simulink model "exampl_Storage_strat_enhanced_R2019a"  (R2019a)
settings: Solver=ode45  StartTime=0.0  StopTime=3*3600-2  RelTol=1e-3  EnableMultiTasking=on
undefined symbols (not defined in the file): path_carnot
libraries: carnot x59, simulink x10
(part 1 of 2)
settings Model: Creator=drhf  LastModifiedBy=P41573
settings DataIOCC: LimitDataPoints=on  SaveFormat=Array  ReturnWorkspaceOutputs=off
settings OptimizationCC: ExpressionDepthLimit=2147483647  LifeSpan=inf
settings DebuggingCC: UnderspecifiedInitializationDetection=Classic  MergeDetectMultiDrivingBlocksExec=none  SolverPrmCheckMsg=warning  StateNameClashWarn=warning  SFUnexpectedBacktrackingDiag=warning  SFNoUnconditionalDefaultTransitionDiag=warning  SFExecutionAtInitializationDiag=none  ArithmeticOperatorsInVariantConditions=warning
settings HardwareCC: ProdBitPerPointer=32  ProdBitPerSizeT=32  ProdBitPerPtrDiffT=32  ProdLargestAtomicFloat=None  ProdIntDivRoundTo=Undefined  ProdEndianess=Unspecified  ProdWordSize=32  ProdHWDeviceType=32-bit Generic
settings ModelReferenceCC: PropagateSignalLabelsOutOfModel=off
settings SFSimCC: SimUseLocalCustomCode=off
settings RTWCC: RTWUseLocalCustomCode=off
settings CodeAppCC: StateflowObjectComments=on
settings GRTTargetCC: TargetLangStandard=C89/C90 (ANSI)  GeneratePreprocessorConditionals=Disable all  CombineOutputUpdateFcns=off  GRTInterface=on
settings ConfigComp: CovMetricSettings=dw  CovHtmlReporting=on  CovSaveCumulativeToWorkspaceVar=on  CovSaveSingleToWorkspaceVar=on  CovExternalEMLEnable=off

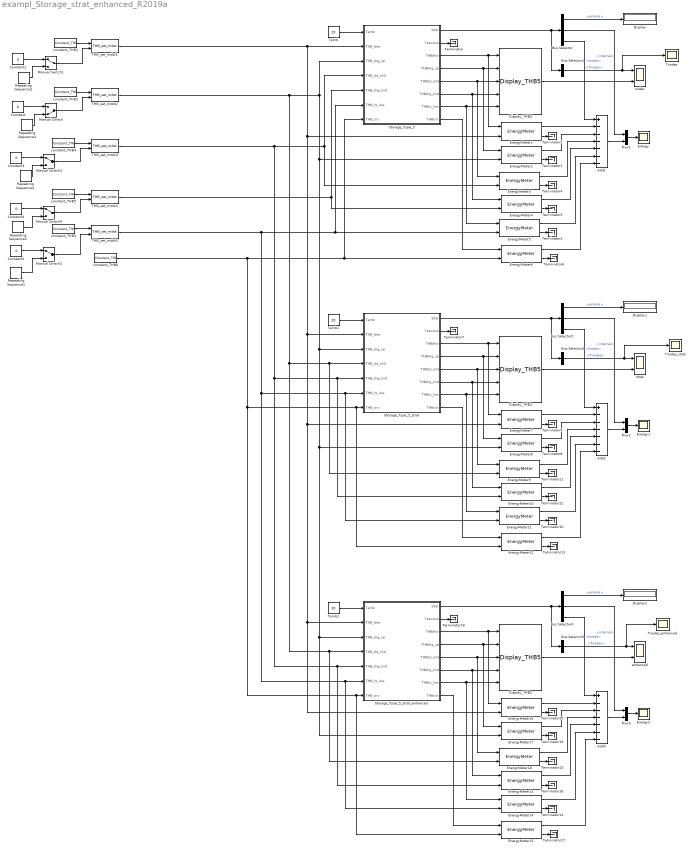
== system exampl_Storage_strat_enhanced_R2019a ==
  Add1 : Sum  Inputs=+------
  Add2 : Sum  Inputs=+------
  Add3 : Sum  Inputs=+------
  Bus Selector : BusSelector  OutputSignals=volume,energy.internal,energy.losses
  Bus Selector1 : BusSelector  OutputSignals=Tnodes
  Bus Selector2 : BusSelector  OutputSignals=volume,energy.internal,energy.losses
  Bus Selector3 : BusSelector  OutputSignals=Tnodes
  Bus Selector4 : BusSelector  OutputSignals=volume,energy.internal,energy.losses
  Bus Selector5 : BusSelector  OutputSignals=Tnodes
  Constant{,1..4} (5 alike) : Constant  Value=0
  Display : Display
  Display1 : Display
  Display2 : Display
  Display_THB1 : carnot/Outputs/Display_THB5  t=off  m=on  p=off  id=off  mix=off  d=off
      settings: SourceProductName=Carnot
  Display_THB2 : carnot/Outputs/Display_THB5  t=off  m=on  p=off  id=off  mix=off  d=off
      settings: SourceProductName=Carnot
  Display_THB5 : carnot/Outputs/Display_THB5  t=off  m=on  p=off  id=off  mix=off  d=off
      settings: SourceProductName=Carnot
  Energy : Scope
  Energy1 : Scope
  Energy2 : Scope
  EnergyMeter{1..18} (18 alike) : carnot/Control/EnergyMeter
      settings: SourceProductName=Carnot
  Manual Switch : ManualSwitch  CurrentSetting=0
  Manual Switch{1..4} (4 alike) : ManualSwitch
  Mux1 : Mux  Inputs=2
  Mux2 : Mux  Inputs=2
  Mux3 : Mux  Inputs=2
  Repeating Sequence1 : simulink/Sources/Repeating Sequence  rep_seq_t=[ 0 3600 3600+eps(3600) 7200 7200+eps(7200) 10800]  rep_seq_y=[ 0.12 0.12 0.11+0*eps(3600) 0.11 0.05+0*eps(7200) 0.05]
  Repeating Sequence2 : simulink/Sources/Repeating Sequence  rep_seq_t=[ 0 3600 3600+eps(3600) 7200 7200+eps(7200) 10440 10440+eps(10440) 11160]  rep_seq_y=[ 0 0 0.05+0*eps(3600) 0.05 0.2+0*eps(7200) 0.2 0+0*eps(10440) 0]
  Repeating Sequence3 : simulink/Sources/Repeating Sequence  rep_seq_t=[ 0 3600 3600+eps(3600) 7200 7200+eps(7200) 10800]  rep_seq_y=[ 0 0 0.1+0*eps(3600) 0.1 0.15+0*eps(7200) 0.15]
  Repeating Sequence4 : simulink/Sources/Repeating Sequence  rep_seq_t=[ 0 3600 3600+eps(3600) 7200 7200+eps(7200) 10800]  rep_seq_y=[ 0.11 0.11 0.1+0*eps(3600) 0.1 0.11+0*eps(7200) 0.11]
  Repeating Sequence5 : simulink/Sources/Repeating Sequence  rep_seq_t=[ 0 3600 3600+eps(3600) 7200 7200+eps(7200) 10800]  rep_seq_y=[ 0.12 0.12 0+0*eps(3600) 0 0.05+0*eps(7200) 0.05]
  Storage_Type_5 : Subsystem  AncestorBlock=carnot/Storage/Thermal/Storage_Type_5  mask(Combi-storage for hot water production and heating){t0=[10:5:55], hgt=1.8108, stgtype=5, tini=[10 15 20 25 30 35 40 45 50 55], mpts=[1 2 3 4 5 6 7 8 9 10], PathName=fullfile(path_carnot('libsl'),'Storage','Thermal','Storage_Type_5','parameter_set'), FileName='<user defined>', userPath=off, userParam=on, uwall=1, ubot=1, utop=1, axcond=1, volume=0.8, dia=0.75, standing=standing cylinder, nodes=10, mpoints=10, Tsensor=[0.2 0.5 0.7], pipe3inlet=1, pipe3outlet=0.6, pipe3dia=0.05, pipe1inlet=0.55, pipe1outlet=0.45, pipe1dia=0.05, hx1inlet=0.4, hx1outlet=0, hx1dia=0.03, hx1uac=200, hx1uam=0.15, hx1uat=0.6, hx1dplin=20, hx1dpqua=20, pipe2inlet=0.45, pipe2outlet=0.55, pipe2dia=0.05, hx2inlet=0, hx2outlet=1, hx2dia=0.025, hx2uac=450, hx2uam=0.4, hx2uat=0.8, hx2dplin=200, hx2dpqua=200, hx3inlet=0.9, hx3outlet=1, hx3dia=0.01, hx3uac=100, hx3uam=0, hx3uat=0, hx3dplin=10, hx3dpqua=10}
      mask prompts: t0 "Initial temperature (vector or scalar) in °C"; hgt "Height of storage in m"; stgtype "Storage Type (0..5)"; tini "Start temperatures of nodes in °C"; mpts "Index to measured nodes"; PathName "Path"; FileName "Parameter set"; userPath "Edit path and name of parameter set"; userParam "User defined parameters"; uwall "Heat transfer coefficient to ambient [W/m²K]"; ubot "Heat transfer coefficient to ambient bottom [W/m²K]"; utop "Heat transfer coefficient to ambient top [W/m²K]"; axcond "Effective thermal conductivity [W/m/K]"; volume "Volume [m³]"; dia "Diameter [m]"; standing "Position"; nodes "Number of nodes"; mpoints "Number of node temperatures (for display)"; Tsensor "Temperature sensor position (0..1, 0 = bottom, 1 = top)"; pipe3inlet "relative height of inlet, range from 0 (= bottom) to 1 (= top)"; pipe3outlet "relative height of outlet, range from 0 (= bottom) to 1 (= top)"; pipe3dia "Diameter of pipe in m"; pipe1inlet "relative height of inlet, range from 0 (= bottom) to 1 (= top)"; pipe1outlet "relative height of outlet, range from 0 (= bottom) to 1 (= top)"; pipe1dia "Diameter of pipe in m"; hx1inlet "relative height of inlet"; hx1outlet "relative height of outlet"; hx1dia "Diameter of HX pipe [m]"; hx1uac "uac: heat transfer coefficient [W/K /(kg/s) /(°C)]"; hx1uam "uam: massflow dependent heat transfer [-]"; hx1uat "uat: temperature difference dependent heat transfer [-]"; hx1dplin "pressure drop linear in mdot [Pa*s/kg]"; hx1dpqua "pressure drop quadratic in mdot [Pa*s²/kg²]"; pipe2inlet "relative height of inlet, range from 0 (= bottom) to 1 (= top)"; pipe2outlet "relative height of outlet, range from 0 (= bottom) to 1 (= top)"; pipe2dia "Diameter of pipe in m"; hx2inlet "relative height of inlet"; hx2outlet "relative height of outlet"; hx2dia "Diameter of HX pipe [m]"; hx2uac "uac: heat transfer coefficient [W/K /(kg/s) /(°C)]"; hx2uam "uam: massflow dependent heat transfer [-]"; hx2uat "uat: temperature difference dependent heat transfer [-]"; hx2dplin "pressure drop linear in mdot [Pa*s/kg]"; hx2dpqua "pressure drop quadratic in mdot [Pa*s²/kg²]"; hx3inlet "relative height of inlet"; hx3outlet "relative height of outlet"; hx3dia "Diameter of HX pipe [m]"; hx3uac "uac: constant heat transfer coefficient [W/K]"; hx3uam "uam: massflow dependent heat transfer [W*s/(K*kg)]"; hx3uat "uat: temperature difference dependent heat transfer [W/K²]"; hx3dplin "Pressure drop coefficient dplin [Pa/(kg/s)]"; hx3dpqua "Pressure drop coefficient dpqua [Pa/(kg/s)²]"
      mask help:
      | Combi-storage for hot water production and heating.  The backup heater for the heating circuit is working on the storage.
      | The storage model has the following components (with their typical position):
      | - one solar heat exchanger (lower part)
      | - one hot water heat exchanger (total height)
      | - one hot water circulation heat exchanger (top part)
      | - one pipe connection for the heating circuit (middle part)
      | - one pipe connection for the backup heater (middle part)
      | - one pipe connection to heat the storage for hot water production (upper part )
      mask init:
      | [ok, param] = CarnotCallbacks_StorageConf('SetParam',stgtype,gcbh,PathName,FileName);
      mask Help: web(fullfile(path_carnot('help'),'Storage_Type_N.html'),'-helpbrowser')
      mask TypeOptions hgt: HX_EN12977_1/hgt | HX_EN12977_2/hgt | HX_EN12977_3/hgt | Pipe_Connection_1/hgt | Pipe_Connection_2_old/hgt | Pipe_Connection_3/hgt | Pipe_Connection_3_enhanced/hgt | Pipe_Connection_3_strat/hgt
      mask TypeOptions stgtype: CreateSdat/stgtype
      mask TypeOptions tini: sfun_storageTnodes/tini
      mask TypeOptions mpts: select_T/Indices
      mask Callback userPath: [ok, param] = CarnotCallbacks_StorageConf('UserEdit',5,gcbh);
      mask Callback userParam: [ok, param] = CarnotCallbacks_StorageConf('UserEdit',5,gcbh);
      mask TypeOptions uwall: sfun_storageTnodes/uloss
      mask TypeOptions ubot: sfun_storageTnodes/ubot
      mask TypeOptions utop: sfun_storageTnodes/utop
      mask TypeOptions axcond: sfun_storageTnodes/cond
      mask TypeOptions volume: sfun_storageTnodes/volume | CreateSdat/volume
      mask TypeOptions dia: sfun_storageTnodes/dia | Pipe_Connection_1/dstg | Pipe_Connection_2_old/dstg | Pipe_Connection_3/dstg | Pipe_Connection_3_strat/dstg
      mask TypeOptions standing: sfun_storageTnodes/standing
      mask TypeOptions nodes: sfun_storageTnodes/nodes | select_T/InputPortWidth | HX_EN12977_1/nodes | HX_EN12977_2/nodes | HX_EN12977_3/nodes | Pipe_Connection_1/nodes | Pipe_Connection_2_old/nodes | Pipe_Connection_3/nodes | Pipe_Connection_3_enhanced/nodes | Pipe_Connection_3_strat/nodes
      mask TypeOptions Tsensor: T_Sensor_Surface/pos
      mask TypeOptions pipe3inlet: Pipe_Connection_3/h_in | Pipe_Connection_3_strat/h_in | Pipe_Connection_3_enhanced/h_in
      mask TypeOptions pipe3outlet: Pipe_Connection_3/h_out | Pipe_Connection_3_enhanced/h_out | Pipe_Connection_3_strat/h_out
      mask TypeOptions pipe3dia: Pipe_Connection_3/dpipe | Pipe_Connection_3_enhanced/dia | Pipe_Connection_3_strat/dpipe
      mask TypeOptions pipe1inlet: Pipe_Connection_1/h_in
      mask TypeOptions pipe1outlet: Pipe_Connection_1/h_out
      mask TypeOptions pipe1dia: Pipe_Connection_1/dpipe
      mask TypeOptions hx1inlet: HX_EN12977_1/h_in
      mask TypeOptions hx1outlet: HX_EN12977_1/h_out
      mask TypeOptions hx1dia: HX_EN12977_1/dia
      mask TypeOptions hx1uac: HX_EN12977_1/ua0
      mask TypeOptions hx1uam: HX_EN12977_1/uam
      mask TypeOptions hx1uat: HX_EN12977_1/uat
      mask TypeOptions hx1dplin: HX_EN12977_1/dplin
      mask TypeOptions hx1dpqua: HX_EN12977_1/dpqua
      mask TypeOptions pipe2inlet: Pipe_Connection_2_old/h_in
      mask TypeOptions pipe2outlet: Pipe_Connection_2_old/h_out
      mask TypeOptions pipe2dia: Pipe_Connection_2_old/dpipe
      mask TypeOptions hx2inlet: HX_EN12977_2/h_in
      mask TypeOptions hx2outlet: HX_EN12977_2/h_out
      mask TypeOptions hx2dia: HX_EN12977_2/dia
      mask TypeOptions hx2uac: HX_EN12977_2/ua0
      mask TypeOptions hx2uam: HX_EN12977_2/uam
      mask TypeOptions hx2uat: HX_EN12977_2/uat
      mask TypeOptions hx2dplin: HX_EN12977_2/dplin
      mask TypeOptions hx2dpqua: HX_EN12977_2/dpqua
      mask TypeOptions hx3inlet: HX_EN12977_3/h_in
      mask TypeOptions hx3outlet: HX_EN12977_3/h_out
      mask TypeOptions hx3dia: HX_EN12977_3/dia
      mask TypeOptions hx3uac: HX_EN12977_3/ua0
      mask TypeOptions hx3uam: HX_EN12977_3/uam
      mask TypeOptions hx3uat: HX_EN12977_3/uat
      mask TypeOptions hx3dplin: HX_EN12977_3/dplin
      mask TypeOptions hx3dpqua: HX_EN12977_3/dpqua
      mask DialogControl Container14 Prompt: Infos
      mask DialogControl ParameterGroupVar Prompt: Picking a parameter set
      mask DialogControl Control3 Prompt: Carnot public data
      mask DialogControl Control3 Callback: [ok, file] = CarnotCallbacks_StorageConf('GetFilename',5,gcbh,'public');
      mask DialogControl Control4 Prompt: Carnot internal data
      mask DialogControl Control4 Callback: [ok, file] = CarnotCallbacks_StorageConf('GetFilename',5,gcbh,'internal');
      mask DialogControl Control2 Prompt: Selected path
      mask DialogControl Control2 Callback: [ok, file] = CarnotCallbacks_StorageConf('GetFilename',5,gcbh,'selected');
      mask DialogControl Container4 Prompt: Parameter values
      mask DialogControl Container6 Prompt: Storage
      mask DialogControl Container8 Prompt: Connections
      mask DialogControl Container9 Prompt: Charging pipe (upper part)
      mask DialogControl Container10 Prompt: Charging pipe (middle part)
      mask DialogControl Container11 Prompt: Charging HX (lower part)
      mask DialogControl Container12 Prompt: Discharging pipe (house heating)
      mask DialogControl Container13 Prompt: HX DHW
      mask DialogControl Container16 Prompt: HX DHW circulation
      mask DialogControl Control6 Prompt: Save in Carnot internal data
      mask DialogControl Control6 Callback: [ok, param] = CarnotCallbacks_StorageConf('SaveFilename',5,gcbh,'internal','STG');
      mask DialogControl Control5 Prompt: Save in selected path
      mask DialogControl Control5 Callback: [ok, param] = CarnotCallbacks_StorageConf('SaveFilename',5,gcbh,'selected','STG');
      mask Display:
      | % user defined picture file
      | namestr = ['Storage_Type_', num2str(get_param(gcb,'stgtype'))];
      | picfile = fullfile(path_carnot('intlibsl'), 'Storage','Thermal', ...
      |     namestr,'parameter_set', [namestr, '.jpg']);
      | 
      | % show internal picture if defined
      | pic = false;
      | if  ~BlockIsInCarnotLibrary       % if not located in library
      |     if exist(picfile, 'file')
      |         image(imread(picfile), [0.3, 0, 0.45, 1])
      |         set_param(gcb, 'BackgroundColor', 'White')
      |         pic = true;
      |     end
      | end
      | 
      | % show public picture
      | if ~pic
      |     set_param(gcb, 'BackgroundColor', 'Red')
      |     plot([36,36,40,50,54,54,50,40,36]/100,[90,50,45,45,50,90,93,93,90]/100, ...
      |         [36,51,40,51,36]/100,[50,50,68,85,85]/100,[36,51,44,51,36]/100, ...
      |         [54,54,56,58,58]/100)
      | end
  Storage_Type_5_strat : Subsystem  AncestorBlock=carnot/Storage/Thermal/Storage_Type_5  mask(Combi-storage for hot water production and heating){t0=[10:5:55], hgt=1.8108, stgtype=5, tini=[10 15 20 25 30 35 40 45 50 55], mpts=[1 2 3 4 5 6 7 8 9 10], PathName=fullfile(path_carnot('libsl'),'Storage','Thermal','Storage_Type_5','parameter_set'), FileName='<user defined>', userPath=off, userParam=on, uwall=1, ubot=1, utop=1, axcond=1, volume=0.8, dia=0.75, standing=standing cylinder, nodes=10, mpoints=10, Tsensor=[0.2 0.5 0.7], pipe3inlet=1, pipe3outlet=0.6, pipe3dia=0.05, pipe1inlet=0.55, pipe1outlet=0.45, pipe1dia=0.05, hx1inlet=0.4, hx1outlet=0, hx1dia=0.03, hx1uac=200, hx1uam=0.15, hx1uat=0.6, hx1dplin=20, hx1dpqua=20, pipe2inlet=0.45, pipe2outlet=0.55, pipe2dia=0.05, hx2inlet=0, hx2outlet=1, hx2dia=0.025, hx2uac=450, hx2uam=0.4, hx2uat=0.8, hx2dplin=200, hx2dpqua=200, hx3inlet=0.9, hx3outlet=1, hx3dia=0.01, hx3uac=100, hx3uam=0, hx3uat=0, hx3dplin=10, hx3dpqua=10}
      mask prompts: t0 "Initial temperature (vector or scalar) in °C"; hgt "Height of storage in m"; stgtype "Storage Type (0..5)"; tini "Start temperatures of nodes in °C"; mpts "Index to measured nodes"; PathName "Path"; FileName "Parameter set"; userPath "Edit path and name of parameter set"; userParam "User defined parameters"; uwall "Heat transfer coefficient to ambient [W/m²K]"; ubot "Heat transfer coefficient to ambient bottom [W/m²K]"; utop "Heat transfer coefficient to ambient top [W/m²K]"; axcond "Effective thermal conductivity [W/m/K]"; volume "Volume [m³]"; dia "Diameter [m]"; standing "Position"; nodes "Number of nodes"; mpoints "Number of node temperatures (for display)"; Tsensor "Temperature sensor position (0..1, 0 = bottom, 1 = top)"; pipe3inlet "relative height of inlet, range from 0 (= bottom) to 1 (= top)"; pipe3outlet "relative height of outlet, range from 0 (= bottom) to 1 (= top)"; pipe3dia "Diameter of pipe in m"; pipe1inlet "relative height of inlet, range from 0 (= bottom) to 1 (= top)"; pipe1outlet "relative height of outlet, range from 0 (= bottom) to 1 (= top)"; pipe1dia "Diameter of pipe in m"; hx1inlet "relative height of inlet"; hx1outlet "relative height of outlet"; hx1dia "Diameter of HX pipe [m]"; hx1uac "uac: heat transfer coefficient [W/K /(kg/s) /(°C)]"; hx1uam "uam: massflow dependent heat transfer [-]"; hx1uat "uat: temperature difference dependent heat transfer [-]"; hx1dplin "pressure drop linear in mdot [Pa*s/kg]"; hx1dpqua "pressure drop quadratic in mdot [Pa*s²/kg²]"; pipe2inlet "relative height of inlet, range from 0 (= bottom) to 1 (= top)"; pipe2outlet "relative height of outlet, range from 0 (= bottom) to 1 (= top)"; pipe2dia "Diameter of pipe in m"; hx2inlet "relative height of inlet"; hx2outlet "relative height of outlet"; hx2dia "Diameter of HX pipe [m]"; hx2uac "uac: heat transfer coefficient [W/K /(kg/s) /(°C)]"; hx2uam "uam: massflow dependent heat transfer [-]"; hx2uat "uat: temperature difference dependent heat transfer [-]"; hx2dplin "pressure drop linear in mdot [Pa*s/kg]"; hx2dpqua "pressure drop quadratic in mdot [Pa*s²/kg²]"; hx3inlet "relative height of inlet"; hx3outlet "relative height of outlet"; hx3dia "Diameter of HX pipe [m]"; hx3uac "uac: constant heat transfer coefficient [W/K]"; hx3uam "uam: massflow dependent heat transfer [W*s/(K*kg)]"; hx3uat "uat: temperature difference dependent heat transfer [W/K²]"; hx3dplin "Pressure drop coefficient dplin [Pa/(kg/s)]"; hx3dpqua "Pressure drop coefficient dpqua [Pa/(kg/s)²]"
      mask help:
      | Combi-storage for hot water production and heating.  The backup heater for the heating circuit is working on the storage.
      | The storage model has the following components (with their typical position):
      | - one solar heat exchanger (lower part)
      | - one hot water heat exchanger (total height)
      | - one hot water circulation heat exchanger (top part)
      | - one pipe connection for the heating circuit (middle part)
      | - one pipe connection for the backup heater (middle part)
      | - one pipe connection to heat the storage for hot water production (upper part )
      mask init:
      | [ok, param] = CarnotCallbacks_StorageConf('SetParam',stgtype,gcbh,PathName,FileName);
      mask Help: web(fullfile(path_carnot('help'),'Storage_Type_N.html'),'-helpbrowser')
      mask TypeOptions hgt: HX_EN12977_1/hgt | HX_EN12977_2/hgt | HX_EN12977_3/hgt | Pipe_Connection_1/hgt | Pipe_Connection_2_old/hgt | Pipe_Connection_3/hgt | Pipe_Connection_3_enhanced/hgt | Pipe_Connection_3_strat/hgt
      mask TypeOptions stgtype: CreateSdat/stgtype
      mask TypeOptions tini: sfun_storageTnodes/tini
      mask TypeOptions mpts: select_T/Indices
      mask Callback userPath: [ok, param] = CarnotCallbacks_StorageConf('UserEdit',5,gcbh);
      mask Callback userParam: [ok, param] = CarnotCallbacks_StorageConf('UserEdit',5,gcbh);
      mask TypeOptions uwall: sfun_storageTnodes/uloss
      mask TypeOptions ubot: sfun_storageTnodes/ubot
      mask TypeOptions utop: sfun_storageTnodes/utop
      mask TypeOptions axcond: sfun_storageTnodes/cond
      mask TypeOptions volume: sfun_storageTnodes/volume | CreateSdat/volume
      mask TypeOptions dia: sfun_storageTnodes/dia | Pipe_Connection_1/dstg | Pipe_Connection_2_old/dstg | Pipe_Connection_3/dstg | Pipe_Connection_3_strat/dstg
      mask TypeOptions standing: sfun_storageTnodes/standing
      mask TypeOptions nodes: sfun_storageTnodes/nodes | select_T/InputPortWidth | HX_EN12977_1/nodes | HX_EN12977_2/nodes | HX_EN12977_3/nodes | Pipe_Connection_1/nodes | Pipe_Connection_2_old/nodes | Pipe_Connection_3/nodes | Pipe_Connection_3_enhanced/nodes | Pipe_Connection_3_strat/nodes
      mask TypeOptions Tsensor: T_Sensor_Surface/pos
      mask TypeOptions pipe3inlet: Pipe_Connection_3/h_in | Pipe_Connection_3_strat/h_in | Pipe_Connection_3_enhanced/h_in
      mask TypeOptions pipe3outlet: Pipe_Connection_3/h_out | Pipe_Connection_3_enhanced/h_out | Pipe_Connection_3_strat/h_out
      mask TypeOptions pipe3dia: Pipe_Connection_3/dpipe | Pipe_Connection_3_enhanced/dia | Pipe_Connection_3_strat/dpipe
      mask TypeOptions pipe1inlet: Pipe_Connection_1/h_in
      mask TypeOptions pipe1outlet: Pipe_Connection_1/h_out
      mask TypeOptions pipe1dia: Pipe_Connection_1/dpipe
      mask TypeOptions hx1inlet: HX_EN12977_1/h_in
      mask TypeOptions hx1outlet: HX_EN12977_1/h_out
      mask TypeOptions hx1dia: HX_EN12977_1/dia
      mask TypeOptions hx1uac: HX_EN12977_1/ua0
      mask TypeOptions hx1uam: HX_EN12977_1/uam
      mask TypeOptions hx1uat: HX_EN12977_1/uat
      mask TypeOptions hx1dplin: HX_EN12977_1/dplin
      mask TypeOptions hx1dpqua: HX_EN12977_1/dpqua
      mask TypeOptions pipe2inlet: Pipe_Connection_2_old/h_in
      mask TypeOptions pipe2outlet: Pipe_Connection_2_old/h_out
      mask TypeOptions pipe2dia: Pipe_Connection_2_old/dpipe
      mask TypeOptions hx2inlet: HX_EN12977_2/h_in
      mask TypeOptions hx2outlet: HX_EN12977_2/h_out
      mask TypeOptions hx2dia: HX_EN12977_2/dia
      mask TypeOptions hx2uac: HX_EN12977_2/ua0
      mask TypeOptions hx2uam: HX_EN12977_2/uam
      mask TypeOptions hx2uat: HX_EN12977_2/uat
      mask TypeOptions hx2dplin: HX_EN12977_2/dplin
      mask TypeOptions hx2dpqua: HX_EN12977_2/dpqua
      mask TypeOptions hx3inlet: HX_EN12977_3/h_in
      mask TypeOptions hx3outlet: HX_EN12977_3/h_out
      mask TypeOptions hx3dia: HX_EN12977_3/dia
      mask TypeOptions hx3uac: HX_EN12977_3/ua0
      mask TypeOptions hx3uam: HX_EN12977_3/uam
      mask TypeOptions hx3uat: HX_EN12977_3/uat
      mask TypeOptions hx3dplin: HX_EN12977_3/dplin
      mask TypeOptions hx3dpqua: HX_EN12977_3/dpqua
      mask DialogControl Container14 Prompt: Infos
      mask DialogControl ParameterGroupVar Prompt: Picking a parameter set
      mask DialogControl Control3 Prompt: Carnot public data
      mask DialogControl Control3 Callback: [ok, file] = CarnotCallbacks_StorageConf('GetFilename',5,gcbh,'public');
      mask DialogControl Control4 Prompt: Carnot internal data
      mask DialogControl Control4 Callback: [ok, file] = CarnotCallbacks_StorageConf('GetFilename',5,gcbh,'internal');
      mask DialogControl Control2 Prompt: Selected path
      mask DialogControl Control2 Callback: [ok, file] = CarnotCallbacks_StorageConf('GetFilename',5,gcbh,'selected');
      mask DialogControl Container4 Prompt: Parameter values
      mask DialogControl Container6 Prompt: Storage
      mask DialogControl Container8 Prompt: Connections
      mask DialogControl Container9 Prompt: Charging pipe (upper part)
      mask DialogControl Container10 Prompt: Charging pipe (middle part)
      mask DialogControl Container11 Prompt: Charging HX (lower part)
      mask DialogControl Container12 Prompt: Discharging pipe (house heating)
      mask DialogControl Container13 Prompt: HX DHW
      mask DialogControl Container16 Prompt: HX DHW circulation
      mask DialogControl Control6 Prompt: Save in Carnot internal data
      mask DialogControl Control6 Callback: [ok, param] = CarnotCallbacks_StorageConf('SaveFilename',5,gcbh,'internal','STG');
      mask DialogControl Control5 Prompt: Save in selected path
      mask DialogControl Control5 Callback: [ok, param] = CarnotCallbacks_StorageConf('SaveFilename',5,gcbh,'selected','STG');
      mask Display:
      | % user defined picture file
      | namestr = ['Storage_Type_', num2str(get_param(gcb,'stgtype'))];
      | picfile = fullfile(path_carnot('intlibsl'), 'Storage','Thermal', ...
      |     namestr,'parameter_set', [namestr, '.jpg']);
      | 
      | % show internal picture if defined
      | pic = false;
      | if  ~BlockIsInCarnotLibrary       % if not located in library
      |     if exist(picfile, 'file')
      |         image(imread(picfile), [0.3, 0, 0.45, 1])
      |         set_param(gcb, 'BackgroundColor', 'White')
      |         pic = true;
      |     end
      | end
      | 
      | % show public picture
      | if ~pic
      |     set_param(gcb, 'BackgroundColor', 'Red')
      |     plot([36,36,40,50,54,54,50,40,36]/100,[90,50,45,45,50,90,93,93,90]/100, ...
      |         [36,51,40,51,36]/100,[50,50,68,85,85]/100,[36,51,44,51,36]/100, ...
      |         [54,54,56,58,58]/100)
      | end
  Storage_Type_5_strat_enhanced : Subsystem  AncestorBlock=carnot/Storage/Thermal/Storage_Type_5  mask(Combi-storage for hot water production and heating){t0=[10:5:55], hgt=1.8108, stgtype=5, tini=[10 15 20 25 30 35 40 45 50 55], mpts=[1 2 3 4 5 6 7 8 9 10], PathName=fullfile(path_carnot('libsl'),'Storage','Thermal','Storage_Type_5','parameter_set'), FileName='<user defined>', userPath=off, userParam=on, uwall=1, ubot=1, utop=1, axcond=1, volume=0.8, dia=0.75, standing=standing cylinder, nodes=10, mpoints=10, Tsensor=[0.2 0.5 0.7], pipe3inlet=1, pipe3outlet=0.6, pipe3dia=0.05, pipe1inlet=0.55, pipe1outlet=0.45, pipe1dia=0.05, hx1inlet=0.4, hx1outlet=0, hx1dia=0.03, hx1uac=200, hx1uam=0.15, hx1uat=0.6, hx1dplin=20, hx1dpqua=20, pipe2inlet=0.45, pipe2outlet=0.55, pipe2dia=0.05, hx2inlet=0, hx2outlet=1, hx2dia=0.025, hx2uac=450, hx2uam=0.4, hx2uat=0.8, hx2dplin=200, hx2dpqua=200, hx3inlet=0.9, hx3outlet=1, hx3dia=0.01, hx3uac=100, hx3uam=0, hx3uat=0, hx3dplin=10, hx3dpqua=10}
      mask prompts: t0 "Initial temperature (vector or scalar) in °C"; hgt "Height of storage in m"; stgtype "Storage Type (0..5)"; tini "Start temperatures of nodes in °C"; mpts "Index to measured nodes"; PathName "Path"; FileName "Parameter set"; userPath "Edit path and name of parameter set"; userParam "User defined parameters"; uwall "Heat transfer coefficient to ambient [W/m²K]"; ubot "Heat transfer coefficient to ambient bottom [W/m²K]"; utop "Heat transfer coefficient to ambient top [W/m²K]"; axcond "Effective thermal conductivity [W/m/K]"; volume "Volume [m³]"; dia "Diameter [m]"; standing "Position"; nodes "Number of nodes"; mpoints "Number of node temperatures (for display)"; Tsensor "Temperature sensor position (0..1, 0 = bottom, 1 = top)"; pipe3inlet "relative height of inlet, range from 0 (= bottom) to 1 (= top)"; pipe3outlet "relative height of outlet, range from 0 (= bottom) to 1 (= top)"; pipe3dia "Diameter of pipe in m"; pipe1inlet "relative height of inlet, range from 0 (= bottom) to 1 (= top)"; pipe1outlet "relative height of outlet, range from 0 (= bottom) to 1 (= top)"; pipe1dia "Diameter of pipe in m"; hx1inlet "relative height of inlet"; hx1outlet "relative height of outlet"; hx1dia "Diameter of HX pipe [m]"; hx1uac "uac: heat transfer coefficient [W/K /(kg/s) /(°C)]"; hx1uam "uam: massflow dependent heat transfer [-]"; hx1uat "uat: temperature difference dependent heat transfer [-]"; hx1dplin "pressure drop linear in mdot [Pa*s/kg]"; hx1dpqua "pressure drop quadratic in mdot [Pa*s²/kg²]"; pipe2inlet "relative height of inlet, range from 0 (= bottom) to 1 (= top)"; pipe2outlet "relative height of outlet, range from 0 (= bottom) to 1 (= top)"; pipe2dia "Diameter of pipe in m"; hx2inlet "relative height of inlet"; hx2outlet "relative height of outlet"; hx2dia "Diameter of HX pipe [m]"; hx2uac "uac: heat transfer coefficient [W/K /(kg/s) /(°C)]"; hx2uam "uam: massflow dependent heat transfer [-]"; hx2uat "uat: temperature difference dependent heat transfer [-]"; hx2dplin "pressure drop linear in mdot [Pa*s/kg]"; hx2dpqua "pressure drop quadratic in mdot [Pa*s²/kg²]"; hx3inlet "relative height of inlet"; hx3outlet "relative height of outlet"; hx3dia "Diameter of HX pipe [m]"; hx3uac "uac: constant heat transfer coefficient [W/K]"; hx3uam "uam: massflow dependent heat transfer [W*s/(K*kg)]"; hx3uat "uat: temperature difference dependent heat transfer [W/K²]"; hx3dplin "Pressure drop coefficient dplin [Pa/(kg/s)]"; hx3dpqua "Pressure drop coefficient dpqua [Pa/(kg/s)²]"
      mask help:
      | Combi-storage for hot water production and heating.  The backup heater for the heating circuit is working on the storage.
      | The storage model has the following components (with their typical position):
      | - one solar heat exchanger (lower part)
      | - one hot water heat exchanger (total height)
      | - one hot water circulation heat exchanger (top part)
      | - one pipe connection for the heating circuit (middle part)
      | - one pipe connection for the backup heater (middle part)
      | - one pipe connection to heat the storage for hot water production (upper part )
      mask init:
      | [ok, param] = CarnotCallbacks_StorageConf('SetParam',stgtype,gcbh,PathName,FileName);
      mask Help: web(fullfile(path_carnot('help'),'Storage_Type_N.html'),'-helpbrowser')
      mask TypeOptions hgt: HX_EN12977_1/hgt | HX_EN12977_2/hgt | HX_EN12977_3/hgt | Pipe_Connection_1/hgt | Pipe_Connection_2_old/hgt | Pipe_Connection_3/hgt | Pipe_Connection_3_enhanced/hgt | Pipe_Connection_3_strat/hgt
      mask TypeOptions stgtype: CreateSdat/stgtype
      mask TypeOptions tini: sfun_storageTnodes/tini
      mask TypeOptions mpts: select_T/Indices
      mask Callback userPath: [ok, param] = CarnotCallbacks_StorageConf('UserEdit',5,gcbh);
      mask Callback userParam: [ok, param] = CarnotCallbacks_StorageConf('UserEdit',5,gcbh);
      mask TypeOptions uwall: sfun_storageTnodes/uloss
      mask TypeOptions ubot: sfun_storageTnodes/ubot
      mask TypeOptions utop: sfun_storageTnodes/utop
      mask TypeOptions axcond: sfun_storageTnodes/cond
      mask TypeOptions volume: sfun_storageTnodes/volume | CreateSdat/volume
      mask TypeOptions dia: sfun_storageTnodes/dia | Pipe_Connection_1/dstg | Pipe_Connection_2_old/dstg | Pipe_Connection_3/dstg | Pipe_Connection_3_strat/dstg
      mask TypeOptions standing: sfun_storageTnodes/standing
      mask TypeOptions nodes: sfun_storageTnodes/nodes | select_T/InputPortWidth | HX_EN12977_1/nodes | HX_EN12977_2/nodes | HX_EN12977_3/nodes | Pipe_Connection_1/nodes | Pipe_Connection_2_old/nodes | Pipe_Connection_3/nodes | Pipe_Connection_3_enhanced/nodes | Pipe_Connection_3_strat/nodes
      mask TypeOptions Tsensor: T_Sensor_Surface/pos
      mask TypeOptions pipe3inlet: Pipe_Connection_3/h_in | Pipe_Connection_3_strat/h_in | Pipe_Connection_3_enhanced/h_in
      mask TypeOptions pipe3outlet: Pipe_Connection_3/h_out | Pipe_Connection_3_enhanced/h_out | Pipe_Connection_3_strat/h_out
      mask TypeOptions pipe3dia: Pipe_Connection_3/dpipe | Pipe_Connection_3_enhanced/dia | Pipe_Connection_3_strat/dpipe
      mask TypeOptions pipe1inlet: Pipe_Connection_1/h_in
      mask TypeOptions pipe1outlet: Pipe_Connection_1/h_out
      mask TypeOptions pipe1dia: Pipe_Connection_1/dpipe
      mask TypeOptions hx1inlet: HX_EN12977_1/h_in
      mask TypeOptions hx1outlet: HX_EN12977_1/h_out
      mask TypeOptions hx1dia: HX_EN12977_1/dia
      mask TypeOptions hx1uac: HX_EN12977_1/ua0
      mask TypeOptions hx1uam: HX_EN12977_1/uam
      mask TypeOptions hx1uat: HX_EN12977_1/uat
      mask TypeOptions hx1dplin: HX_EN12977_1/dplin
      mask TypeOptions hx1dpqua: HX_EN12977_1/dpqua
      mask TypeOptions pipe2inlet: Pipe_Connection_2_old/h_in
      mask TypeOptions pipe2outlet: Pipe_Connection_2_old/h_out
      mask TypeOptions pipe2dia: Pipe_Connection_2_old/dpipe
      mask TypeOptions hx2inlet: HX_EN12977_2/h_in
      mask TypeOptions hx2outlet: HX_EN12977_2/h_out
      mask TypeOptions hx2dia: HX_EN12977_2/dia
      mask TypeOptions hx2uac: HX_EN12977_2/ua0
      mask TypeOptions hx2uam: HX_EN12977_2/uam
      mask TypeOptions hx2uat: HX_EN12977_2/uat
      mask TypeOptions hx2dplin: HX_EN12977_2/dplin
      mask TypeOptions hx2dpqua: HX_EN12977_2/dpqua
      mask TypeOptions hx3inlet: HX_EN12977_3/h_in
      mask TypeOptions hx3outlet: HX_EN12977_3/h_out
      mask TypeOptions hx3dia: HX_EN12977_3/dia
      mask TypeOptions hx3uac: HX_EN12977_3/ua0
      mask TypeOptions hx3uam: HX_EN12977_3/uam
      mask TypeOptions hx3uat: HX_EN12977_3/uat
      mask TypeOptions hx3dplin: HX_EN12977_3/dplin
      mask TypeOptions hx3dpqua: HX_EN12977_3/dpqua
      mask DialogControl Container14 Prompt: Infos
      mask DialogControl ParameterGroupVar Prompt: Picking a parameter set
      mask DialogControl Control3 Prompt: Carnot public data
      mask DialogControl Control3 Callback: [ok, file] = CarnotCallbacks_StorageConf('GetFilename',5,gcbh,'public');
      mask DialogControl Control4 Prompt: Carnot internal data
      mask DialogControl Control4 Callback: [ok, file] = CarnotCallbacks_StorageConf('GetFilename',5,gcbh,'internal');
      mask DialogControl Control2 Prompt: Selected path
      mask DialogControl Control2 Callback: [ok, file] = CarnotCallbacks_StorageConf('GetFilename',5,gcbh,'selected');
      mask DialogControl Container4 Prompt: Parameter values
      mask DialogControl Container6 Prompt: Storage
      mask DialogControl Container8 Prompt: Connections
      mask DialogControl Container9 Prompt: Charging pipe (upper part)
      mask DialogControl Container10 Prompt: Charging pipe (middle part)
      mask DialogControl Container11 Prompt: Charging HX (lower part)
      mask DialogControl Container12 Prompt: Discharging pipe (house heating)
      mask DialogControl Container13 Prompt: HX DHW
      mask DialogControl Container16 Prompt: HX DHW circulation
      mask DialogControl Control6 Prompt: Save in Carnot internal data
      mask DialogControl Control6 Callback: [ok, param] = CarnotCallbacks_StorageConf('SaveFilename',5,gcbh,'internal','STG');
      mask DialogControl Control5 Prompt: Save in selected path
      mask DialogControl Control5 Callback: [ok, param] = CarnotCallbacks_StorageConf('SaveFilename',5,gcbh,'selected','STG');
      mask Display:
      | % user defined picture file
      | namestr = ['Storage_Type_', num2str(get_param(gcb,'stgtype'))];
      | picfile = fullfile(path_carnot('intlibsl'), 'Storage','Thermal', ...
      |     namestr,'parameter_set', [namestr, '.jpg']);
      | 
      | % show internal picture if defined
      | pic = false;
      | if  ~BlockIsInCarnotLibrary       % if not located in library
      |     if exist(picfile, 'file')
      |         image(imread(picfile), [0.3, 0, 0.45, 1])
      |         set_param(gcb, 'BackgroundColor', 'White')
      |         pic = true;
      |     end
      | end
      | 
      | % show public picture
      | if ~pic
      |     set_param(gcb, 'BackgroundColor', 'Red')
      |     plot([36,36,40,50,54,54,50,40,36]/100,[90,50,45,45,50,90,93,93,90]/100, ...
      |         [36,51,40,51,36]/100,[50,50,68,85,85]/100,[36,51,44,51,36]/100, ...
      |         [54,54,56,58,58]/100)
      | end
  THB_set_mdot{1..5} (5 alike) : carnot/Source/Simple/THB_set_mdot
      settings: SourceProductName=Carnot
  Tamb : Constant  Value=20
  Tamb1 : Constant  Value=20
  Tamb2 : Constant  Value=20
  Terminator{,1..20} (21 alike) : Terminator
  Tnodes : Scope
  Tnodes_enhanced : Scope
  Tnodes_strat : Scope
  constant_THB1 : carnot/Source/Simple/Constant_THB  t=15  mdot=0*100/3600  p=1e5  mID=Full Pressure Drop with Static Height  fluid=Water  mix=0  mix2=0  mix3=0  dia=0.02  hgt=0
      settings: SourceProductName=Carnot
  constant_THB2 : carnot/Source/Simple/Constant_THB  t=35  mdot=100/3600  p=1e5  mID=Full Pressure Drop with Static Height  fluid=Water  mix=0  mix2=0  mix3=0  dia=0.02  hgt=0
      settings: SourceProductName=Carnot
  constant_THB3 : carnot/Source/Simple/Constant_THB  t=40  mdot=100/3600  p=1e5  mID=Full Pressure Drop with Static Height  fluid=Water  mix=0  mix2=0  mix3=0  dia=0.02  hgt=0
      settings: SourceProductName=Carnot
  constant_THB4 : carnot/Source/Simple/Constant_THB  t=30  mdot=100/3600  p=1e5  mID=Full Pressure Drop with Static Height  fluid=Water  mix=0  mix2=0  mix3=0  dia=0.02  hgt=0
      settings: SourceProductName=Carnot
  constant_THB5 : carnot/Source/Simple/Constant_THB  t=40  mdot=100/3600  p=1e5  mID=Full Pressure Drop with Static Height  fluid=Water  mix=0  mix2=0  mix3=0  dia=0.02  hgt=0
      settings: SourceProductName=Carnot
  constant_THB6 : carnot/Source/Simple/Constant_THB  t=40  mdot=0  p=1e5  mID=Full Pressure Drop with Static Height  fluid=Water  mix=0  mix2=0  mix3=0  dia=0.02  hgt=0
      settings: SourceProductName=Carnot
  enhanced : Scope  NumInputPorts=2
  nodes : Scope  NumInputPorts=2
  strat : Scope  NumInputPorts=2
  wires:
  Bus Selector/2 -> Mux1/1  "<internal>"
  Tamb/1 -> Storage_Type_5/1(Tamb)
  Storage_Type_5/1(Sdat) -> Bus Selector1/1, Bus Selector/1
  Storage_Type_5/3(THBdhw) -> EnergyMeter1/1, Display_THB5/1
  Storage_Type_5/4(THBchg_up) -> EnergyMeter2/1, Display_THB5/2
  Display_THB5/1 -> nodes/2
  Mux1/1 -> Energy/1
  EnergyMeter2/2 -> Terminator1/1
  constant_THB1/1 -> THB_set_mdot1/1
  constant_THB2/1 -> THB_set_mdot2/1
  Manual Switch1/1 -> THB_set_mdot1/2
  Manual Switch/1 -> THB_set_mdot2/2
  Constant/1 -> Manual Switch/1
  Repeating Sequence3/1 -> Manual Switch/2
  Constant1/1 -> Manual Switch1/1
  Repeating Sequence2/1 -> Manual Switch1/2
  EnergyMeter1/2 -> Terminator2/1
  Add1/1 -> Mux1/2
  EnergyMeter2/1 -> Add1/3
  EnergyMeter1/1 -> Add1/2
  constant_THB3/1 -> THB_set_mdot5/1
  Manual Switch2/1 -> THB_set_mdot5/2
  Constant2/1 -> Manual Switch2/1
  Repeating Sequence1/1 -> Manual Switch2/2
  EnergyMeter5/2 -> Terminator3/1
  Storage_Type_5/5(THBdis_mid) -> EnergyMeter3/1, Display_THB5/3
  constant_THB4/1 -> THB_set_mdot3/1
  Manual Switch3/1 -> THB_set_mdot3/2
  Constant3/1 -> Manual Switch3/1
  Repeating Sequence4/1 -> Manual Switch3/2
  EnergyMeter3/2 -> Terminator4/1
  Storage_Type_5/7(THBhx_low) -> EnergyMeter5/1, Display_THB5/5
  constant_THB5/1 -> THB_set_mdot4/1
  Manual Switch4/1 -> THB_set_mdot4/2
  Constant4/1 -> Manual Switch4/1
  Repeating Sequence5/1 -> Manual Switch4/2
  THB_set_mdot4/1 -> Storage_Type_5/5(THB_chg_mid), EnergyMeter4/2
  Storage_Type_5/6(THBchg_mid) -> EnergyMeter4/1, Display_THB5/4
  EnergyMeter5/1 -> Add1/6
  Bus Selector/3 -> Add1/1  "<losses>"
  EnergyMeter3/1 -> Add1/4
  EnergyMeter4/2 -> Terminator5/1
  EnergyMeter4/1 -> Add1/5
  Bus Selector/1 -> Display/1  "<volume>"
  EnergyMeter6/2 -> Terminator6/1
  Storage_Type_5/8(THBcirc) -> EnergyMeter6/1
  EnergyMeter6/1 -> Add1/7
  Storage_Type_5/2(Tsensors) -> Terminator/1
  Bus Selector1/1 -> Tnodes/1, nodes/1  "<Tnodes>"
  Storage_Type_5_strat/2(Tsensors) -> Terminator7/1
  EnergyMeter11/2 -> Terminator10/1
  EnergyMeter7/1 -> Add2/2
  Bus Selector3/1 -> Tnodes_strat/1, strat/1  "<Tnodes>"
  EnergyMeter10/1 -> Add2/5
  EnergyMeter9/2 -> Terminator11/1
  Storage_Type_5_strat/8(THBcirc) -> EnergyMeter12/1
  EnergyMeter12/1 -> Add2/7
  Bus Selector2/3 -> Add2/1  "<losses>"
  EnergyMeter11/1 -> Add2/6
  EnergyMeter9/1 -> Add2/4
  EnergyMeter10/2 -> Terminator12/1
  Storage_Type_5_strat/7(THBhx_low) -> EnergyMeter11/1, Display_THB1/5
  Storage_Type_5_strat/5(THBdis_mid) -> EnergyMeter9/1, Display_THB1/3
  Add2/1 -> Mux2/2
  Storage_Type_5_strat/6(THBchg_mid) -> EnergyMeter10/1, Display_THB1/4
  Storage_Type_5_strat/3(THBdhw) -> EnergyMeter7/1, Display_THB1/1
  EnergyMeter12/2 -> Terminator13/1
  EnergyMeter7/2 -> Terminator9/1
  Bus Selector2/2 -> Mux2/1  "<internal>"
  EnergyMeter8/2 -> Terminator8/1
  Storage_Type_5_strat/4(THBchg_up) -> EnergyMeter8/1, Display_THB1/2
  Mux2/1 -> Energy1/1
  Bus Selector2/1 -> Display1/1  "<volume>"
  EnergyMeter8/1 -> Add2/3
  Display_THB1/1 -> strat/2
  Storage_Type_5_strat/1(Sdat) -> Bus Selector3/1, Bus Selector2/1
  Tamb1/1 -> Storage_Type_5_strat/1(Tamb)
  Tamb2/1 -> Storage_Type_5_strat_enhanced/1(Tamb)
  Storage_Type_5_strat_enhanced/1(Sdat) -> Bus Selector4/1, Bus Selector5/1
  THB_set_mdot1/1 -> Storage_Type_5/2(THB_dhw), EnergyMeter1/2, Storage_Type_5_strat/2(THB_dhw), EnergyMeter16/2, Storage_Type_5_strat_enhanced/2(THB_dhw), EnergyMeter7/2
  Display_THB2/1 -> enhanced/2
  EnergyMeter17/1 -> Add3/3
  THB_set_mdot5/1 -> Storage_Type_5_strat_enhanced/6(THB_hx_low), EnergyMeter14/2, EnergyMeter11/2, Storage_Type_5_strat/6(THB_hx_low), EnergyMeter5/2, Storage_Type_5/6(THB_hx_low)
  Bus Selector4/1 -> Display2/1  "<volume>"
  Mux3/1 -> Energy2/1
  Storage_Type_5_strat_enhanced/4(THBchg_up) -> Display_THB2/2, EnergyMeter17/1
  EnergyMeter17/2 -> Terminator19/1
  Bus Selector4/2 -> Mux3/1  "<internal>"
  EnergyMeter16/2 -> Terminator20/1
  EnergyMeter15/2 -> Terminator17/1
  Storage_Type_5_strat_enhanced/3(THBdhw) -> Display_THB2/1, EnergyMeter16/1
  Storage_Type_5_strat_enhanced/6(THBchg_mid) -> Display_THB2/4, EnergyMeter13/1
  Add3/1 -> Mux3/2
  THB_set_mdot3/1 -> EnergyMeter13/2, Storage_Type_5_strat_enhanced/5(THB_chg_mid), Storage_Type_5_strat/5(THB_chg_mid), EnergyMeter10/2, Storage_Type_5/4(THB_dis_mid), EnergyMeter3/2
  THB_set_mdot2/1 -> Storage_Type_5_strat_enhanced/4(THB_dis_mid), EnergyMeter18/2, EnergyMeter9/2, Storage_Type_5_strat/4(THB_dis_mid), Storage_Type_5_strat_enhanced/3(THB_chg_up), EnergyMeter17/2, EnergyMeter8/2, Storage_Type_5_strat/3(THB_chg_up), EnergyMeter2/2, Storage_Type_5/3(THB_chg_up)
  Storage_Type_5_strat_enhanced/5(THBdis_mid) -> Display_THB2/3, EnergyMeter18/1
  Storage_Type_5_strat_enhanced/7(THBhx_low) -> Display_THB2/5, EnergyMeter14/1
  EnergyMeter13/2 -> Terminator16/1
  EnergyMeter18/1 -> Add3/4
  EnergyMeter14/1 -> Add3/6
  Bus Selector4/3 -> Add3/1  "<losses>"
  EnergyMeter15/1 -> Add3/7
  Storage_Type_5_strat_enhanced/8(THBcirc) -> EnergyMeter15/1
  EnergyMeter18/2 -> Terminator15/1
  EnergyMeter13/1 -> Add3/5
  Bus Selector5/1 -> Tnodes_enhanced/1, enhanced/1  "<Tnodes>"
  EnergyMeter16/1 -> Add3/2
  EnergyMeter14/2 -> Terminator14/1
  Storage_Type_5_strat_enhanced/2(Tsensors) -> Terminator18/1
  constant_THB6/1 -> EnergyMeter6/2, Storage_Type_5/7(THB_circ), Storage_Type_5_strat_enhanced/7(THB_circ), EnergyMeter15/2, EnergyMeter12/2, Storage_Type_5_strat/7(THB_circ)

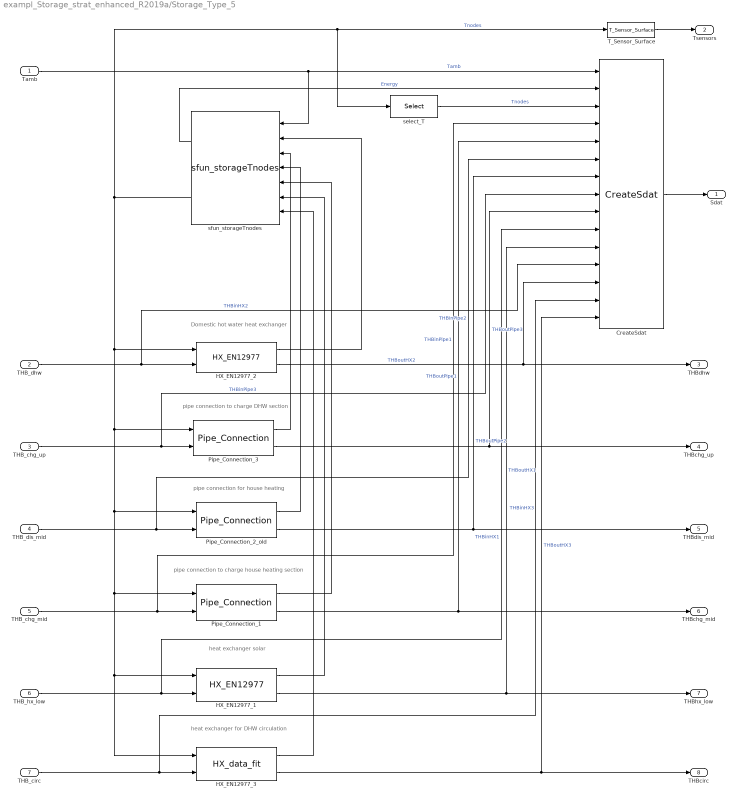
== system exampl_Storage_strat_enhanced_R2019a/Storage_Type_5 ==
  note: heat exchanger for DHW circulation
  note: heat exchanger solar
  note: pipe connection to charge house heating section
  note: pipe connection for house heating
  note: pipe connection to charge DHW section
  note: Domestic hot water heat exchanger
  Tamb : Inport
  THB_dhw : Inport  Port=2
  THB_chg_up : Inport  Port=3
  THB_dis_mid : Inport  Port=4
  THB_chg_mid : Inport  Port=5
  THB_hx_low : Inport  Port=6
  THB_circ : Inport  Port=7
  CreateSdat : carnot/Basic/Thermal_Models/CreateSdat  volume=volume  stgtype=stgtype
      settings: SourceProductName=Carnot
  HX_EN12977_1 : carnot/Storage/Thermal/Storage_Ports/HX_EN12977  h_in=hx1inlet  h_out=hx1outlet  hgt=hgt  dia=hx1dia  height=-0.72432  ua0=hx1uac  uam=hx1uam  uat=hx1uat  dplin=hx1dplin  dpqua=hx1dpqua  nodes=nodes
      settings: SourceProductName=Carnot
  HX_EN12977_2 : carnot/Storage/Thermal/Storage_Ports/HX_EN12977  h_in=hx2inlet  h_out=hx2outlet  hgt=hgt  dia=hx2dia  height=1.8108  ua0=hx2uac  uam=hx2uam  uat=hx2uat  dplin=hx2dplin  dpqua=hx2dpqua  nodes=nodes
      settings: SourceProductName=Carnot
  HX_EN12977_3 : carnot/Storage/Thermal/Storage_Ports/HX_data_fit  h_in=hx3inlet  h_out=hx3outlet  hgt=hgt  dia=hx3dia  height=0.18108  ua0=hx3uac  uam=hx3uam  uat=hx3uat  dplin=hx3dplin  dpqua=hx3dpqua  nodes=nodes
      settings: SourceProductName=Carnot
  Pipe_Connection_1 : carnot/Storage/Thermal/Storage_Ports/Pipe_Connection  h_in=pipe1inlet  h_out=pipe1outlet  hgt=hgt  dpipe=pipe1dia  dstg=dia  height=-0.18108  nodes=nodes
      settings: SourceProductName=Carnot
  Pipe_Connection_2_old : carnot/Storage/Thermal/Storage_Ports/Pipe_Connection  h_in=pipe2inlet  h_out=pipe2outlet  hgt=hgt  dpipe=pipe2dia  dstg=dia  height=0.18108  nodes=nodes
      settings: SourceProductName=Carnot
  Pipe_Connection_3 : carnot/Storage/Thermal/Storage_Ports/Pipe_Connection  h_in=pipe3inlet  h_out=pipe3outlet  hgt=hgt  dpipe=pipe3dia  dstg=dia  height=-0.72432  nodes=nodes
      settings: SourceProductName=Carnot
  T_Sensor_Surface : carnot/Control/T_Sensor_Surface  pos=Tsensor  tdel=10  t0=mean(tini)
      settings: SourceProductName=Carnot
  select_T : Selector  InputPortWidth=nodes  IndexOptions=Index vector (dialog)  Indices=[1 2 3 4 5 6 7 8 9 10]  OutputSizes=1
  sfun_storageTnodes : carnot/Basic/Thermal_Models/sfun_storageTnodes  uloss=uwall  ubot=ubot  utop=utop  cond=axcond  volume=volume  dia=dia  standing=standing cylinder  tini=tini  nodes=nodes  nconnect=6  elimthermocline=2  condinvtc=1e5
      settings: SourceProductName=Carnot
  Sdat : Outport
  Tsensors : Outport  Port=2
  THBdhw : Outport  Port=3
  THBchg_up : Outport  Port=4
  THBdis_mid : Outport  Port=5
  THBchg_mid : Outport  Port=6
  THBhx_low : Outport  Port=7
  THBcirc : Outport  Port=8
  wires:
  sfun_storageTnodes/1 -> CreateSdat/2  "Energy"
  Pipe_Connection_1/2 -> CreateSdat/5, THBchg_mid/1  "THBoutPipe1"
  Pipe_Connection_1/1 -> sfun_storageTnodes/5
  THB_chg_mid/1 -> Pipe_Connection_1/2, CreateSdat/4  "THBinPipe1"
  HX_EN12977_1/1 -> sfun_storageTnodes/6
  Pipe_Connection_2_old/2 -> CreateSdat/7, THBdis_mid/1  "THBoutPipe2"
  Pipe_Connection_2_old/1 -> sfun_storageTnodes/4
  THB_dis_mid/1 -> Pipe_Connection_2_old/2, CreateSdat/6  "THBinPipe2"
  Tamb/1 -> CreateSdat/1, sfun_storageTnodes/1  "Tamb"
  THB_dhw/1 -> HX_EN12977_2/2, CreateSdat/12  "THBinHX2"
  HX_EN12977_2/2 -> CreateSdat/13, THBdhw/1  "THBoutHX2"
  HX_EN12977_2/1 -> sfun_storageTnodes/2
  select_T/1 -> CreateSdat/3  "Tnodes"
  sfun_storageTnodes/2 -> select_T/1, T_Sensor_Surface/1, Pipe_Connection_3/1, HX_EN12977_3/1, HX_EN12977_1/1, Pipe_Connection_1/1, Pipe_Connection_2_old/1, HX_EN12977_2/1  "Tnodes"
  CreateSdat/1 -> Sdat/1
  THB_chg_up/1 -> Pipe_Connection_3/2, CreateSdat/8  "THBinPipe3"
  Pipe_Connection_3/2 -> CreateSdat/9, THBchg_up/1  "THBoutPipe3"
  Pipe_Connection_3/1 -> sfun_storageTnodes/3
  THB_hx_low/1 -> HX_EN12977_1/2, CreateSdat/10  "THBinHX1"
  HX_EN12977_1/2 -> CreateSdat/11, THBhx_low/1  "THBoutHX1"
  T_Sensor_Surface/1 -> Tsensors/1
  THB_circ/1 -> HX_EN12977_3/2, CreateSdat/14  "THBinHX3"
  HX_EN12977_3/1 -> sfun_storageTnodes/7
  HX_EN12977_3/2 -> CreateSdat/15, THBcirc/1  "THBoutHX3"
